simulink model "stm32f4discovery_audio_equalizer_part3"  (R2016b)
settings: Solver=ode3  StartTime=0.0  StopTime=Inf  RelTol=1e-3  EnableMultiTasking=on
PreLoadFcn:
  | % disp(['Running PreLoadFcn Callback for ' bdroot]);
  | 
  | dspparameq_data
  | 
  | % disp('PreLoadFcn Callback Complete')
undefined symbols (not defined in the file): bits, CoeffsMatrix1, CoeffsMatrix2, CoeffsMatrix3, dfilt
libraries: stm32f4lib x2, dsparch4 x1
CloseFcn:
  | % disp(['Running CloseFcn Callback for ' bdroot]);
  | 
  | % Delete parameters
  | clear Fs CoeffsMatrix1 CoeffsMatrix2  CoeffsMatrix3
  | clear coeffsMatrix1   coeffsMatrix2   coeffsMatrix3
  | clear in out
settings Model: SimulationMode=external  ExtModeTrigDuration=1  Creator=The MathWorks, Inc.  LastModifiedBy=bhavya
settings DataIOCC: LimitDataPoints=on  SaveFormat=Array
settings OptimizationCC: BlockReduction=off  BooleanDataType=off  LifeSpan=1  MaxStackSize=64
settings DebuggingCC: SaveWithParameterizedLinksMsg=none  UnderspecifiedInitializationDetection=Classic  MergeDetectMultiDrivingBlocksExec=none  SignalResolutionControl=TryResolveAllWithWarning  ParameterPrecisionLossMsg=none  AllowSymbolicDim=off  SFUnexpectedBacktrackingDiag=warning  SFNoUnconditionalDefaultTransitionDiag=warning  SFExecutionAtInitializationDiag=none
settings HardwareCC: ProdBitPerPointer=32  ProdBitPerSizeT=32  ProdBitPerPtrDiffT=32  ProdLargestAtomicInteger=Long  ProdLargestAtomicFloat=Double  ProdWordSize=32  ProdHWDeviceType=ARM Compatible->ARM Cortex  TargetLargestAtomicInteger=Long  TargetLargestAtomicFloat=Double  TargetEndianess=LittleEndian  TargetHWDeviceType=ARM Compatible->ARM Cortex
settings ModelReferenceCC: PropagateSignalLabelsOutOfModel=off
settings RTWCC: SystemTargetFile=ert.tlc  HardwareBoard=STM32F4-Discovery  TLCOptions=-aInlineSetEventsForThisBaseRateFcn=TLC_FALSE -aSuppressMultiTaskScheduler=TLC_FALSE -aRateBasedStepFcn=1  TemplateMakefile=ert_default_tmf  Description=Embedded Coder  Toolchain=GNU Tools for ARM Embedded Processors
settings CodeAppCC: IgnoreCustomStorageClasses=off
settings ERTTargetCC: CodeReplacementLibrary=ARM Cortex-M  ConvertIfToSwitch=off  SuppressUnreachableDefaultCases=off
settings ConfigComp: CovMetricSettings=dw  CovHtmlReporting=on  CovSaveCumulativeToWorkspaceVar=on  CovSaveSingleToWorkspaceVar=on  CovExternalEMLEnable=off  CovSFcnEnable=off

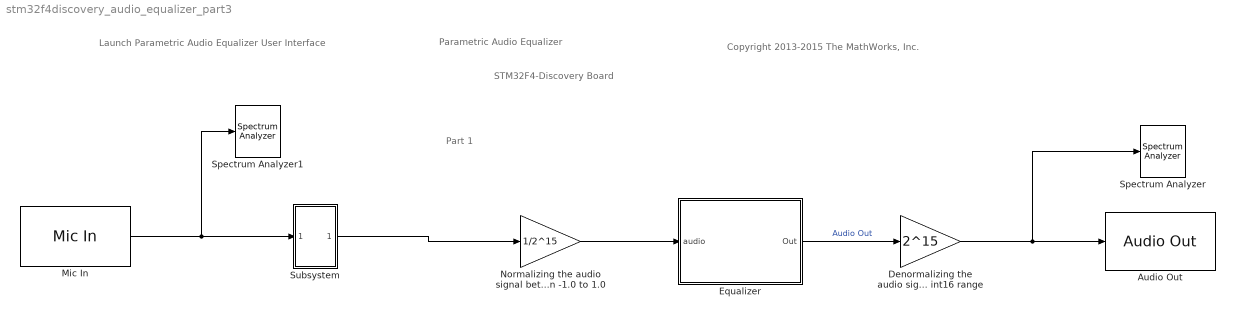
== system stm32f4discovery_audio_equalizer_part3 ==
  note: Part 1
  note: Parametric Audio Equalizer
  note: Copyright 2013-2015 The MathWorks, Inc.
  note: STM32F4-Discovery Board
  note: Launch Parametric Audio Equalizer User Interface
  Audio Out : stm32f4lib/Audio Out  sampling_rate_freq=44100
  Denormalizing the audio signal to int16 range : Gain  Gain=2^15  ParamDataTypeStr=single  OutDataTypeStr=int16  SaturateOnIntegerOverflow=on
  Equalizer : Subsystem  TreatAsAtomicUnit=on  mask{Fc1=300.0, BW1=300.0, G1=3.0, Fc2=1000.0, BW2=700.0, G2=-2.0, Fc3=3000.0, BW3=500.0, G3=2.0}
      mask prompts: Fc1 "Center Frequency 1"; BW1 "Bandwidth 1"; G1 "Gain 1"; Fc2 "Center Frequency 2"; BW2 "Bandwidth 2"; G2 "Gain 2"; Fc3 "Center Frequency 3"; BW3 "Bandwidth 3"; G3 "Gain 3"
      mask Callback Fc1: paramEQtoBiquad(eval(get_param('stm32f4discovery_audio_equalizer/Equalizer','Fc1')) , 1 , 'stm32f4discovery_audio_equalizer')
      mask Callback BW1: paramEQtoBiquad(eval(get_param('stm32f4discovery_audio_equalizer/Equalizer','BW1')) , 2 , 'stm32f4discovery_audio_equalizer')
      mask Callback G1: paramEQtoBiquad(eval(get_param('stm32f4discovery_audio_equalizer/Equalizer','G1')) , 3 , 'stm32f4discovery_audio_equalizer')
      mask Callback Fc2: paramEQtoBiquad(eval(get_param('stm32f4discovery_audio_equalizer/Equalizer','Fc2')) , 4 , 'stm32f4discovery_audio_equalizer')
      mask Callback BW2: paramEQtoBiquad(eval(get_param('stm32f4discovery_audio_equalizer/Equalizer','BW2')) , 5 , 'stm32f4discovery_audio_equalizer')
      mask Callback G2: paramEQtoBiquad(eval(get_param('stm32f4discovery_audio_equalizer/Equalizer','G2')) , 6 , 'stm32f4discovery_audio_equalizer')
      mask Callback Fc3: paramEQtoBiquad(eval(get_param('stm32f4discovery_audio_equalizer/Equalizer','Fc3')) , 7 , 'stm32f4discovery_audio_equalizer')
      mask Callback BW3: paramEQtoBiquad(eval(get_param('stm32f4discovery_audio_equalizer/Equalizer','BW3')) , 8 , 'stm32f4discovery_audio_equalizer')
      mask Callback G3: paramEQtoBiquad(eval(get_param('stm32f4discovery_audio_equalizer/Equalizer','G3')) , 9 , 'stm32f4discovery_audio_equalizer')
      mask Display: disp(sprintf('Parametric\nAudio\nEqualizer'))
  Mic In : stm32f4lib/Mic In  sampling_rate_freq=16000  bit_resolution=16-bits  samples_per_frame=44.1*20  inherit_sample_time=off  sample_time=44.1*20/16000
  Normalizing the audio signal between -1.0 to 1.0 : Gain  Gain=1/2^15  ParamDataTypeStr=single  OutDataTypeStr=single
  Spectrum Analyzer : SpectrumAnalyzer
  Spectrum Analyzer1 : SpectrumAnalyzer
  Subsystem : Subsystem
  wires:
  Equalizer/1(Out) -> Denormalizing the audio signal to int16 range/1  "Audio Out"
  Denormalizing the audio signal to int16 range/1 -> Spectrum Analyzer/1, Audio Out/1
  Normalizing the audio signal between -1.0 to 1.0/1 -> Equalizer/1(audio)
  Mic In/1 -> Spectrum Analyzer1/1, Subsystem/1(In1)
  Subsystem/1(Out1) -> Normalizing the audio signal between -1.0 to 1.0/1

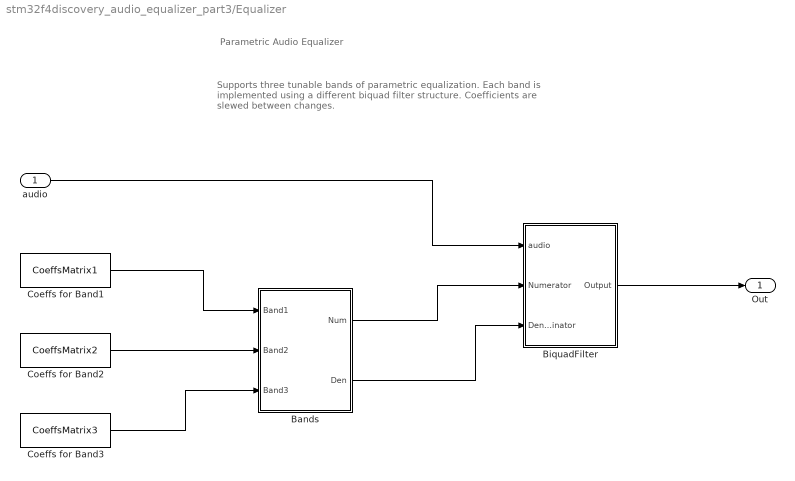
== system stm32f4discovery_audio_equalizer_part3/Equalizer ==
  note: Parametric Audio Equalizer
  note: Supports three tunable bands of parametric equalization.
      | Each band is implemented using a different biquad filter structure.
      | Coefficients are slewed between changes.
  audio : Inport
  Bands : Subsystem  TreatAsAtomicUnit=on
      settings: RTWSystemCode=Nonreusable function
  BiquadFilter : Subsystem  TreatAsAtomicUnit=on
      settings: RTWSystemCode=Nonreusable function
  Coeffs for Band1 : Constant  Value=CoeffsMatrix1  VectorParams1D=off  OutDataTypeStr=single
  Coeffs for Band2 : Constant  Value=CoeffsMatrix2  VectorParams1D=off  OutDataTypeStr=single
  Coeffs for Band3 : Constant  Value=CoeffsMatrix3  VectorParams1D=off  OutDataTypeStr=single
  Out : Outport
  wires:
  audio/1 -> BiquadFilter/1(audio)
  Coeffs for Band1/1 -> Bands/1(Band1)
  Coeffs for Band2/1 -> Bands/2(Band2)
  Coeffs for Band3/1 -> Bands/3(Band3)
  BiquadFilter/1(Output) -> Out/1
  Bands/1(Num) -> BiquadFilter/2(Numerator)
  Bands/2(Den) -> BiquadFilter/3(Denominator)

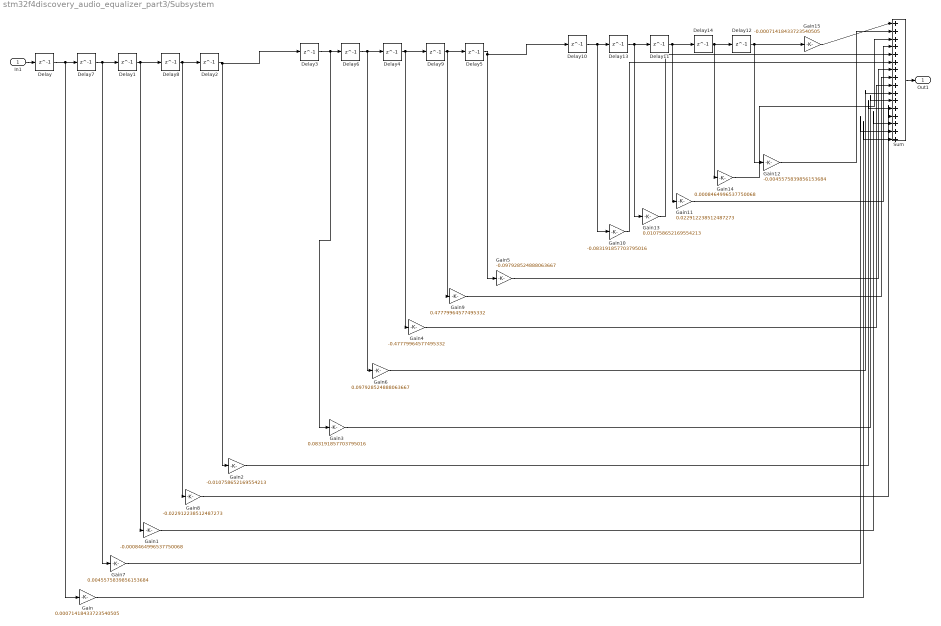
== system stm32f4discovery_audio_equalizer_part3/Subsystem ==
  In1 : Inport
  Delay{,1..14} (15 alike) : Delay  DelayLength=1  InitialCondition=0  InputProcessing=Columns as channels (frame based)
  Gain : Gain  Gain=0.00071418433723540505
  Gain1 : Gain  Gain=-0.0008464996537750068
  Gain10 : Gain  Gain=-0.083191857703795016
  Gain11 : Gain  Gain=0.022912238512487273
  Gain12 : Gain  Gain=-0.0045575839856153684
  Gain13 : Gain  Gain=0.010758652169554213
  Gain14 : Gain  Gain=0.0008464996537750068
  Gain15 : Gain  Gain=-0.00071418433723540505
  Gain2 : Gain  Gain=-0.010758652169554213
  Gain3 : Gain  Gain=0.083191857703795016
  Gain4 : Gain  Gain=-0.47779964577495332
  Gain5 : Gain  Gain=-0.097928524888063667
  Gain6 : Gain  Gain=0.097928524888063667
  Gain7 : Gain  Gain=0.0045575839856153684
  Gain8 : Gain  Gain=-0.022912238512487273
  Gain9 : Gain  Gain=0.47779964577495332
  Sum : Sum  Inputs=|++++++++++++++++
  Out1 : Outport
  wires:
  Gain4/1 -> Sum/9
  Gain2/1 -> Sum/12
  Gain3/1 -> Sum/11
  Gain5/1 -> Sum/7
  Gain13/1 -> Sum/5
  Gain8/1 -> Sum/13
  Gain10/1 -> Sum/6
  Gain1/1 -> Sum/14
  Gain11/1 -> Sum/4
  Gain6/1 -> Sum/10
  Gain12/1 -> Sum/2
  Delay/1 -> Delay7/1, Gain/1
  Delay2/1 -> Delay3/1, Gain2/1
  Delay1/1 -> Delay8/1, Gain1/1
  Delay8/1 -> Delay2/1, Gain8/1
  Delay7/1 -> Delay1/1, Gain7/1
  Delay3/1 -> Delay6/1, Gain3/1
  Delay4/1 -> Delay9/1, Gain4/1
  Delay9/1 -> Delay5/1, Gain9/1
  Delay5/1 -> Delay10/1, Gain5/1
  Delay6/1 -> Delay4/1, Gain6/1
  Gain/1 -> Sum/16
  Gain14/1 -> Sum/3
  In1/1 -> Delay/1
  Sum/1 -> Out1/1
  Gain7/1 -> Sum/15
  Delay12/1 -> Gain15/1, Gain12/1
  Delay13/1 -> Delay11/1, Gain13/1
  Delay14/1 -> Delay12/1, Gain14/1
  Delay10/1 -> Delay13/1, Gain10/1
  Delay11/1 -> Delay14/1, Gain11/1
  Gain9/1 -> Sum/8
  Gain15/1 -> Sum/1

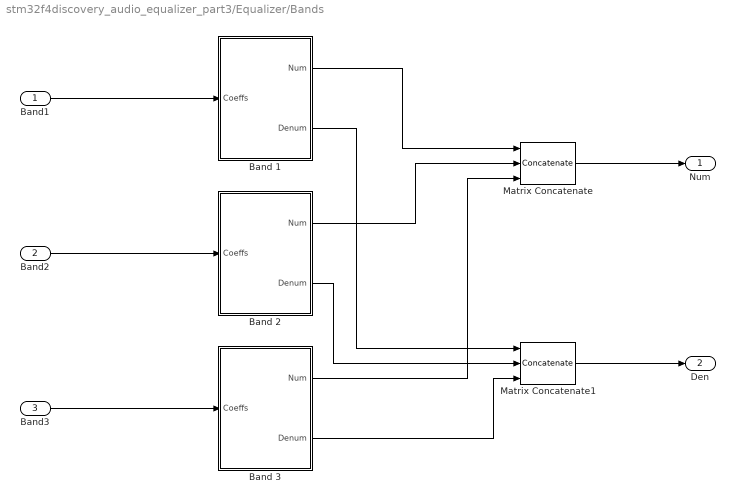
== system stm32f4discovery_audio_equalizer_part3/Equalizer/Bands ==
  Band1 : Inport
  Band2 : Inport  Port=2
  Band3 : Inport  Port=3
  Band 1 : Subsystem  TreatAsAtomicUnit=on
      settings: RTWSystemCode=Nonreusable function
  Band 2 : Subsystem  TreatAsAtomicUnit=on
      settings: RTWSystemCode=Nonreusable function
  Band 3 : Subsystem  TreatAsAtomicUnit=on
      settings: RTWSystemCode=Nonreusable function
  Matrix Concatenate : Concatenate  NumInputs=3  Mode=Multidimensional array  ConcatenateDimension=2
  Matrix Concatenate1 : Concatenate  NumInputs=3  Mode=Multidimensional array  ConcatenateDimension=2
  Num : Outport
  Den : Outport  Port=2
  wires:
  Band1/1 -> Band 1/1(Coeffs)
  Band2/1 -> Band 2/1(Coeffs)
  Band3/1 -> Band 3/1(Coeffs)
  Band 1/1(Num) -> Matrix Concatenate/1
  Band 2/1(Num) -> Matrix Concatenate/2
  Band 3/1(Num) -> Matrix Concatenate/3
  Band 1/2(Denum) -> Matrix Concatenate1/1
  Band 2/2(Denum) -> Matrix Concatenate1/2
  Band 3/2(Denum) -> Matrix Concatenate1/3
  Matrix Concatenate1/1 -> Den/1
  Matrix Concatenate/1 -> Num/1

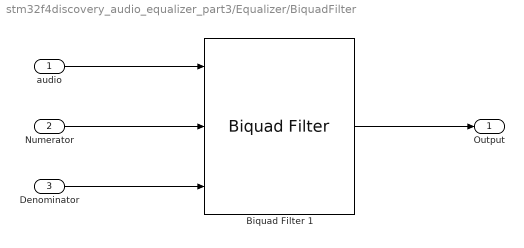
== system stm32f4discovery_audio_equalizer_part3/Equalizer/BiquadFilter ==
  audio : Inport
  Numerator : Inport  Port=2
  Denominator : Inport  Port=3
  Biquad Filter 1 : dsparch4/Biquad Filter  IIRFiltStruct=Direct form II transposed  CoeffSource=Specify via dialog  BiQuadCoeffs=[1 0.3 0.4 1 0.1 0.2]  a0Flag=Warning  IC=0  ICnum=0  ICden=0  InputProcessing=Columns as channels (frame based)  denAccumFracLength=30  denProdOutputFracLength=30  secondMemoryFracLength=15  roundingMode=Floor  overflowMode=off  ScaleValues=1  optimizeScaleValues=on  ScaleValueMode=Assume all are unity and optimize  scaleValueFracLength=14  FilterSource=Input port(s)  FilterObject=dfilt.df2tsos([1 0.3 0.4],[1 0.1 0.2])
      settings: AttributesFormatString=--------------------------------------\n%<IIRFiltStruct>
  Output : Outport
  wires:
  Biquad Filter 1/1 -> Output/1
  audio/1 -> Biquad Filter 1/1
  Numerator/1 -> Biquad Filter 1/2
  Denominator/1 -> Biquad Filter 1/3

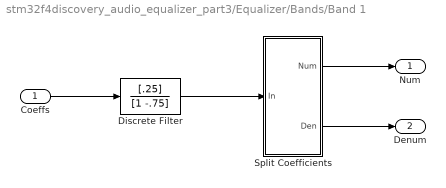
== system stm32f4discovery_audio_equalizer_part3/Equalizer/Bands/Band 1 ==
  Coeffs : Inport
  Discrete Filter : DiscreteFilter  Numerator=[.25]  Denominator=[1 -.75]
  Split Coefficients : Subsystem
  Num : Outport
  Denum : Outport  Port=2
  wires:
  Discrete Filter/1 -> Split Coefficients/1(In)
  Coeffs/1 -> Discrete Filter/1
  Split Coefficients/1(Num) -> Num/1
  Split Coefficients/2(Den) -> Denum/1

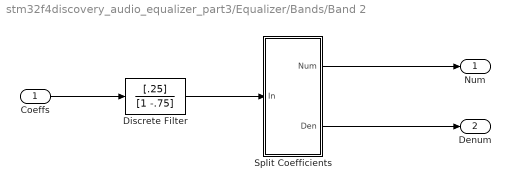
== system stm32f4discovery_audio_equalizer_part3/Equalizer/Bands/Band 2 ==
  Coeffs : Inport
  Discrete Filter : DiscreteFilter  Numerator=[.25]  Denominator=[1 -.75]
  Split Coefficients : Subsystem
  Num : Outport
  Denum : Outport  Port=2
  wires:
  Discrete Filter/1 -> Split Coefficients/1(In)
  Coeffs/1 -> Discrete Filter/1
  Split Coefficients/2(Den) -> Denum/1
  Split Coefficients/1(Num) -> Num/1

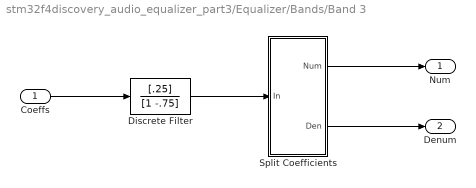
== system stm32f4discovery_audio_equalizer_part3/Equalizer/Bands/Band 3 ==
  Coeffs : Inport
  Discrete Filter : DiscreteFilter  Numerator=[.25]  Denominator=[1 -.75]
  Split Coefficients : Subsystem
  Num : Outport
  Denum : Outport  Port=2
  wires:
  Discrete Filter/1 -> Split Coefficients/1(In)
  Coeffs/1 -> Discrete Filter/1
  Split Coefficients/2(Den) -> Denum/1
  Split Coefficients/1(Num) -> Num/1

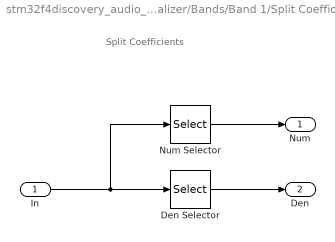
== system stm32f4discovery_audio_equalizer_part3/Equalizer/Bands/Band 1/Split Coefficients ==
  note: Split Coefficients
  In : Inport
  Den Selector : Selector  InputPortWidth=5  IndexOptions=Index vector (dialog)  Indices=[4 5]  OutputSizes=1
  Num Selector : Selector  InputPortWidth=5  IndexOptions=Index vector (dialog)  Indices=[1 2 3]  OutputSizes=1
  Num : Outport
  Den : Outport  Port=2
  wires:
  In/1 -> Num Selector/1, Den Selector/1
  Num Selector/1 -> Num/1
  Den Selector/1 -> Den/1

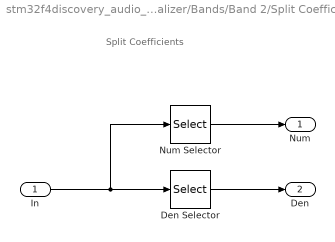
== system stm32f4discovery_audio_equalizer_part3/Equalizer/Bands/Band 2/Split Coefficients ==
  note: Split Coefficients
  In : Inport
  Den Selector : Selector  InputPortWidth=5  IndexOptions=Index vector (dialog)  Indices=[4 5]  OutputSizes=1
  Num Selector : Selector  InputPortWidth=5  IndexOptions=Index vector (dialog)  Indices=[1 2 3]  OutputSizes=1
  Num : Outport
  Den : Outport  Port=2
  wires:
  In/1 -> Num Selector/1, Den Selector/1
  Num Selector/1 -> Num/1
  Den Selector/1 -> Den/1

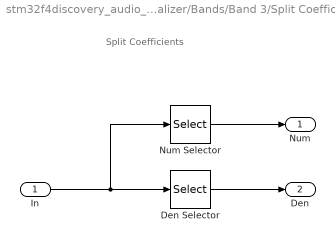
== system stm32f4discovery_audio_equalizer_part3/Equalizer/Bands/Band 3/Split Coefficients ==
  note: Split Coefficients
  In : Inport
  Den Selector : Selector  InputPortWidth=5  IndexOptions=Index vector (dialog)  Indices=[4 5]  OutputSizes=1
  Num Selector : Selector  InputPortWidth=5  IndexOptions=Index vector (dialog)  Indices=[1 2 3]  OutputSizes=1
  Num : Outport
  Den : Outport  Port=2
  wires:
  In/1 -> Num Selector/1, Den Selector/1
  Num Selector/1 -> Num/1
  Den Selector/1 -> Den/1
